simulink model "uav_problem"  (R2024b)
settings: Solver=VariableStepAuto  StartTime=0.0  StopTime=tstop  RelTol=1e-3
values from neighbouring files (symbols this model uses):
  de_max = deg2rad(de_max_deg)    [uav_params_init.m]
  de_min = deg2rad(de_min_deg)    [uav_params_init.m]
  dh = 10    [uav_params_init.m]
  gam0 = 0    [uav_params_init.m]
  h0 = 100    [uav_params_init.m]
  h_step_time = 1    [uav_params_init.m]
  Kd_th = 0.25    [uav_params_init.m]
  Ki_h = 0.01    [uav_params_init.m]
  Ki_th = 0.6    [uav_params_init.m]
  Ki_V = 0.08    [uav_params_init.m]
  Kp_h = 0.04    [uav_params_init.m]
  Kp_th = 2.0    (= 2)    [uav_params_init.m]
  Kp_V = 0.3    [uav_params_init.m]
  N_th = 20    [uav_params_init.m]
  q0 = 0    [uav_params_init.m]
  th0 = alpha0 + gam0    [uav_params_init.m]
  V0 = 20    [uav_params_init.m]
settings Model: Creator=rahulshirishkar  LastModifiedBy=rahulshirishkar

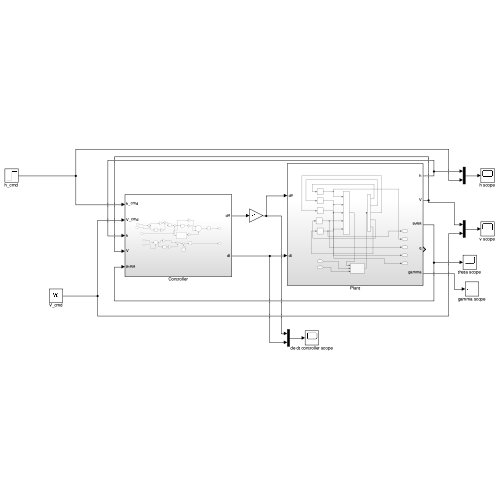
[thumbnail: Simulink's stored preview of the top-level diagram]
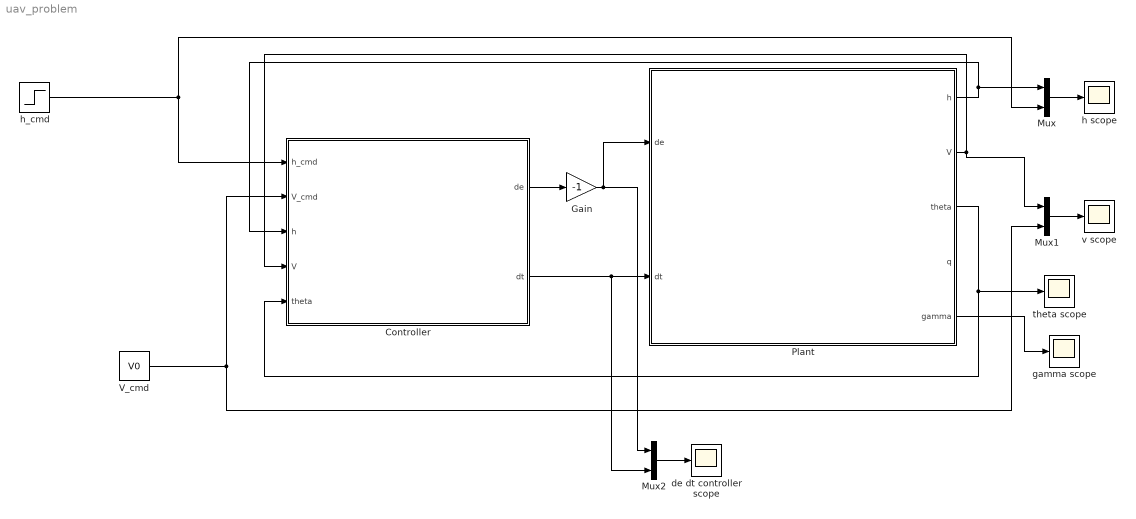
== system uav_problem ==
  Controller : Subsystem
  Gain : Gain  Gain=-1
  Mux : Mux  Inputs=2
  Mux1 : Mux  Inputs=2
  Mux2 : Mux  Inputs=2
  Plant : Subsystem
  V_cmd : Constant  Value=V0
  de dt controller scope : Scope
  gamma scope : Scope
  h scope : Scope
  h_cmd : Step  Time=h_step_time  Before=h0  After=h0+dh  SampleTime=0
  theta scope : Scope
  v scope : Scope
  wires:
  Plant/1(h) -> Mux/1, Controller/3(h)
  Plant/3(theta) -> theta scope/1, Controller/5(theta)
  h_cmd/1 -> Controller/1(h_cmd), Mux/2
  V_cmd/1 -> Mux1/2, Controller/2(V_cmd)
  Mux/1 -> h scope/1
  Plant/2(V) -> Controller/4(V), Mux1/1
  Mux1/1 -> v scope/1
  Mux2/1 -> de dt controller scope/1
  Controller/1(de) -> Gain/1
  Plant/5(gamma) -> gamma scope/1
  Gain/1 -> Plant/1(de), Mux2/1
  Controller/2(dt) -> Plant/2(dt), Mux2/2

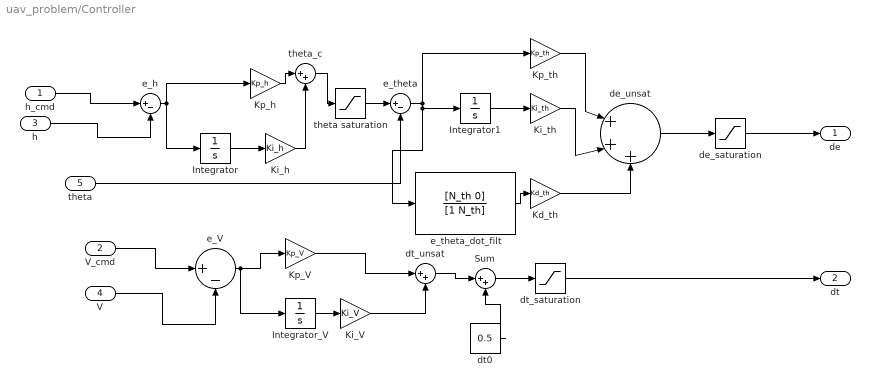
== system uav_problem/Controller ==
  h_cmd : Inport
  V_cmd : Inport  Port=2
  h : Inport  Port=3
  V : Inport  Port=4
  theta : Inport  Port=5
  Integrator : Integrator
  Integrator1 : Integrator
  Integrator_V : Integrator
  Kd_th : Gain  Gain=Kd_th
  Ki_V : Gain  Gain=Ki_V
  Ki_h : Gain  Gain=Ki_h
  Ki_th : Gain  Gain=Ki_th
  Kp_V : Gain  Gain=Kp_V
  Kp_h : Gain  Gain=Kp_h
  Kp_th : Gain  Gain=Kp_th
  Sum : Sum  Inputs=|++
  de_saturation : Saturate  UpperLimit=de_max  LowerLimit=de_min
  de_unsat : Sum  Inputs=|+++
  dt0 : Constant  Value=0.5
  dt_saturation : Saturate  UpperLimit=1  LowerLimit=0
  dt_unsat : Sum  Inputs=|++
  e_V : Sum  Inputs=|+-
  e_h : Sum  Inputs=|+-
  e_theta : Sum  Inputs=|+-
  e_theta_dot_filt : TransferFcn  Numerator=[N_th 0]  Denominator=[1 N_th]
  theta saturation : Saturate  UpperLimit=deg2rad(20)  LowerLimit=deg2rad(-20)
  theta_c : Sum  Inputs=|++
  de : Outport
  dt : Outport  Port=2
  wires:
  h_cmd/1 -> e_h/1
  h/1 -> e_h/2
  e_h/1 -> Integrator/1, Kp_h/1
  Integrator/1 -> Ki_h/1
  Kp_h/1 -> theta_c/1
  Ki_h/1 -> theta_c/2
  theta_c/1 -> theta saturation/1
  theta/1 -> e_theta/2
  e_theta/1 -> e_theta_dot_filt/1, Integrator1/1, Kp_th/1
  Integrator1/1 -> Ki_th/1
  e_theta_dot_filt/1 -> Kd_th/1
  Kp_th/1 -> de_unsat/1
  Ki_th/1 -> de_unsat/2
  Kd_th/1 -> de_unsat/3
  de_unsat/1 -> de_saturation/1
  de_saturation/1 -> de/1
  V_cmd/1 -> e_V/1
  V/1 -> e_V/2
  e_V/1 -> Integrator_V/1, Kp_V/1
  Integrator_V/1 -> Ki_V/1
  Kp_V/1 -> dt_unsat/1
  Ki_V/1 -> dt_unsat/2
  dt_unsat/1 -> Sum/1
  dt_saturation/1 -> dt/1
  dt0/1 -> Sum/2
  Sum/1 -> dt_saturation/1
  theta saturation/1 -> e_theta/1

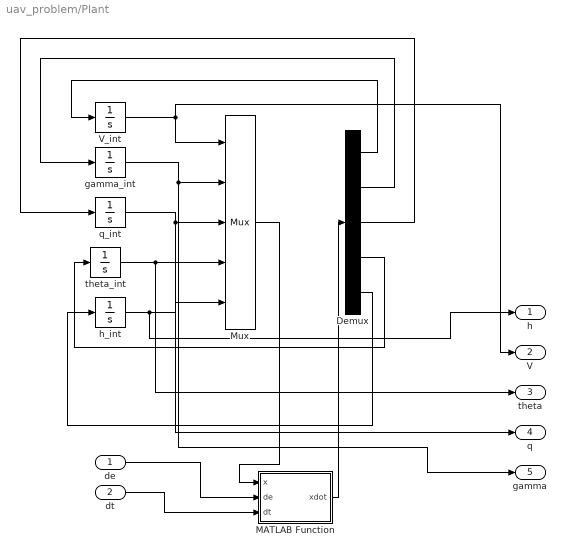
== system uav_problem/Plant ==
  de : Inport
  dt : Inport  Port=2
  Demux : Demux  Outputs=5
  MATLAB Function : MATLAB Function  TreatAsAtomicUnit=on
  Mux : Mux  Inputs=5
  V_int : Integrator  InitialCondition=V0
  gamma_int : Integrator  InitialCondition=gam0
  h_int : Integrator  InitialCondition=h0
  q_int : Integrator  InitialCondition=q0
  theta_int : Integrator  InitialCondition=th0
  h : Outport
  V : Outport  Port=2
  theta : Outport  Port=3
  q : Outport  Port=4
  gamma : Outport  Port=5
  wires:
  V_int/1 -> V/1, Mux/1
  gamma_int/1 -> gamma/1, Mux/2
  q_int/1 -> q/1, Mux/3
  theta_int/1 -> theta/1, Mux/4
  h_int/1 -> h/1, Mux/5
  Mux/1 -> MATLAB Function/1(x)
  de/1 -> MATLAB Function/2(de)
  dt/1 -> MATLAB Function/3(dt)
  MATLAB Function/1(xdot) -> Demux/1
  Demux/1 -> V_int/1
  Demux/2 -> gamma_int/1
  Demux/3 -> q_int/1
  Demux/4 -> theta_int/1
  Demux/5 -> h_int/1

== matlab function uav_problem/Plant/MATLAB Function ==
  data: x input; xdot output; de input; dt input
function xdot = dyn(x,de,dt)
%#codegen

% These are interpreted (not code-generated) functions:
coder.extrinsic('evalin','uav_longitudinal_dyn');

% Pre-allocate so Simulink knows xdot is 5x1
xdot = zeros(5,1);

% Get parameter struct p from base workspace
p = evalin('base','p');

% Call your dynamics – this returns a 5x1 vector
xdot = uav_longitudinal_dyn(x,de,dt,p);
end
